simulink model "week1_problem2"  (R2020a)
settings: Solver=VariableStepAuto  StartTime=0.0  StopTime=10.0  RelTol=1e-3
model workspace (MAT data in the model file):
  b_suspention = 50
  car_weight = 1000
  k_suspention = 50
  k_tire = 20
  tire_weight = 20
settings Model: Creator=hp  LastModifiedBy=hp

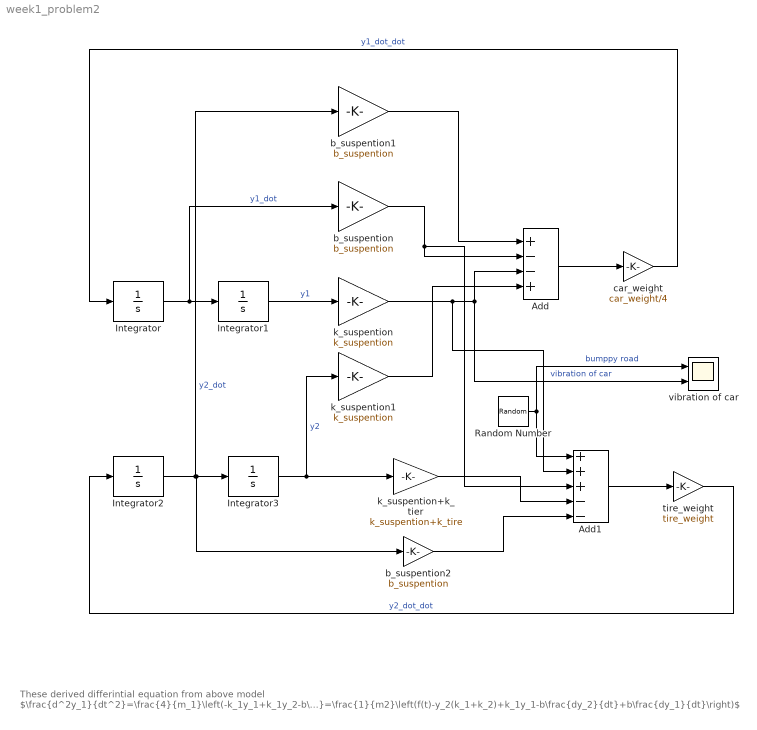
== system week1_problem2 ==
  note: These derived differintial equation from above model
      | $\frac{d^2y_1}{dt^2}=\frac{4}{m_1}\left(-k_1y_1+k_1y_2-b\frac{dy_1}{dt}+b\frac{dy_2}{dt}\right)\\\frac{d^2y_2}{dt^2}=\frac{1}{m2}\left(f(t)-y_2(k_1+k_2)+k_1y_1-b\frac{dy_2}{dt}+b\frac{dy_1}{dt}\right)$
  Add : Sum  Inputs=+--+
  Add1 : Sum  Inputs=+++--
  Integrator{,1..3} (4 alike) : Integrator
  Random Number : RandomNumber  SampleTime=0.1
  b_suspention : Gain  Gain=b_suspention
  b_suspention1 : Gain  Gain=b_suspention
  b_suspention2 : Gain  Gain=b_suspention
  car_weight : Gain  Gain=car_weight/4
  k_suspention : Gain  Gain=k_suspention
  k_suspention+k_tier : Gain  Gain=k_suspention+k_tire
  k_suspention1 : Gain  Gain=k_suspention
  tire_weight : Gain  Gain=tire_weight
  vibration of car : Scope  NumInputPorts=2
  wires:
  k_suspention+k_tier/1 -> Add1/4
  b_suspention/1 -> Add1/3, Add/2
  Add/1 -> car_weight/1
  b_suspention2/1 -> Add1/5
  k_suspention1/1 -> Add/4
  Add1/1 -> tire_weight/1
  Integrator/1 -> b_suspention/1, Integrator1/1  "y1_dot"
  Random Number/1 -> Add1/1, vibration of car/1  "bumppy road"
  Integrator2/1 -> b_suspention1/1, b_suspention2/1, Integrator3/1  "y2_dot"
  b_suspention1/1 -> Add/1
  Integrator1/1 -> k_suspention/1  "y1"
  car_weight/1 -> Integrator/1  "y1_dot_dot"
  k_suspention/1 -> Add1/2, vibration of car/2, Add/3  "vibration of car"
  Integrator3/1 -> k_suspention+k_tier/1, k_suspention1/1  "y2"
  tire_weight/1 -> Integrator2/1  "y2_dot_dot"
